simulink model "Take_off_distance"  (R2021b)
settings: Solver=VariableStepAuto  StartTime=0.0  StopTime=300  RelTol=1e-3
settings Model: Creator=manavbathija  LastModifiedBy=manavbathija
settings SolverCC: AlgebraicLoopSolver=TrustRegion
settings DebuggingCC: SFMachineParentedDataDiag=warning

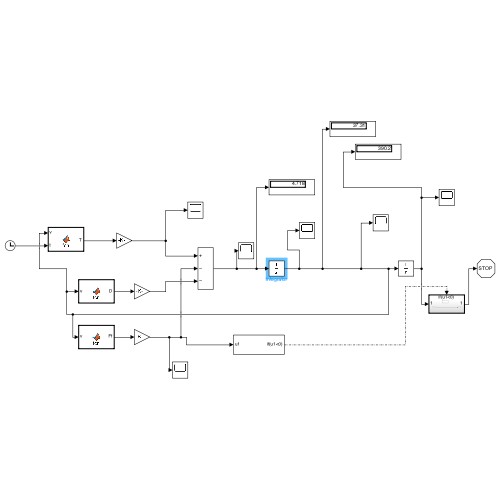
[thumbnail: Simulink's stored preview of the top-level diagram]
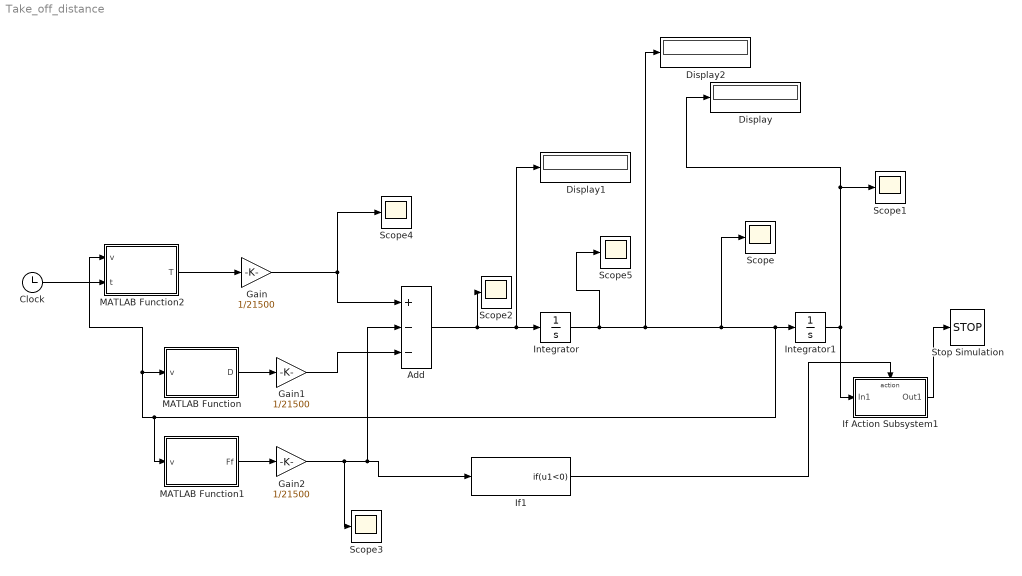
== system Take_off_distance ==
  Add : Sum  Inputs=+--
  Clock : Clock
  Display : Display
  Display1 : Display
  Display2 : Display
  Gain : Gain  Gain=1/21500
  Gain1 : Gain  Gain=1/21500
  Gain2 : Gain  Gain=1/21500
  If Action Subsystem1 : Subsystem  TreatAsAtomicUnit=on
  If1 : If  IfExpression=u1<0  ShowElse=off
  Integrator : Integrator  InitialCondition=.001
  Integrator1 : Integrator
  MATLAB Function : MATLAB Function  TreatAsAtomicUnit=on
  MATLAB Function1 : MATLAB Function  TreatAsAtomicUnit=on
  MATLAB Function2 : MATLAB Function  TreatAsAtomicUnit=on
  Scope{,1..5} (6 alike) : Scope
  Stop Simulation : Stop
  wires:
  Gain/1 -> Scope4/1, Add/1
  MATLAB Function/1(D) -> Gain1/1
  MATLAB Function1/1(Ff) -> Gain2/1
  Gain2/1 -> Scope3/1, Add/2, If1/1
  Add/1 -> Scope2/1, Display1/1, Integrator/1
  Integrator1/1 -> If Action Subsystem1/1(In1), Scope1/1, Display/1
  If Action Subsystem1/1(Out1) -> Stop Simulation/1
  If1/1 -> If Action Subsystem1/Action
  Integrator/1 -> Scope5/1, Display2/1, Integrator1/1, MATLAB Function1/1(v), MATLAB Function2/1(v), MATLAB Function/1(v), Scope/1
  Gain1/1 -> Add/3
  MATLAB Function2/1(T) -> Gain/1
  Clock/1 -> MATLAB Function2/2(t)

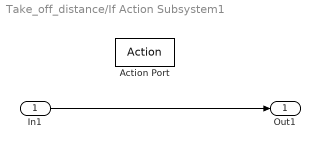
== system Take_off_distance/If Action Subsystem1 ==
  In1 : Inport
  Action Port : ActionPort  ActionPortLabel=if(u1<0)
  Out1 : Outport
  wires:
  In1/1 -> Out1/1

== matlab function Take_off_distance/MATLAB Function ==
  data: v input; D output
function D = fcn(v)

D = 0.5*1.225*v^2*156*(0.04+(1/(pi*8.5*0.7))*2.6^2);

== matlab function Take_off_distance/MATLAB Function2 ==
  data: v input; T output; t input
function T = fcn(v,t)
rpm=1212*t/15;
P=14913*rpm*0.10472;
T= 2*0.8*P/v;

== matlab function Take_off_distance/MATLAB Function1 ==
  data: v input; Ff output
function Ff = fcn(v)
L=0.5*1.225*v^2*156*2.6;
u=0.69;
Ff=u*(35290*9.8-L);
